simulink model "Subsystem"  (R2020b)
settings: Solver=FixedStepAuto  StartTime=0.0  StopTime=10.0  FixedStep=0.001  RelTol=1e-3
values from neighbouring files (symbols this model uses):
  a0 = 1    [Initializing_prob7.m]
  a1 = 1    [Initializing_prob7.m]
  a2 = -1    [Initializing_prob7.m]
  b0 = 1    [Initializing_prob7.m]
  b1 = 2    [Initializing_prob7.m]
  b2 = -1    [Initializing_prob7.m]
settings Model: Creator=Lakshmi  LastModifiedBy=Lakshmi
settings DataIOCC: SaveOutput=off  SaveTime=off

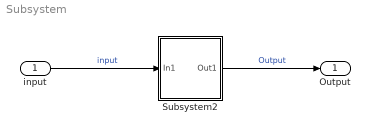
== system Subsystem ==
  input : Inport  OutDataTypeStr=double  PortDimensions=1  SampleTime=[0.001,0]
  Subsystem2 : Subsystem
  Output : Outport  OutDataTypeStr=double  PortDimensions=1  SampleTime=[0.001,0]
  wires:
  input/1 -> Subsystem2/1(In1)  "input"
  Subsystem2/1(Out1) -> Output/1  "Output"

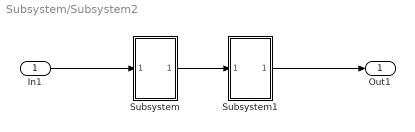
== system Subsystem/Subsystem2 ==
  In1 : Inport
  Subsystem : Subsystem
  Subsystem1 : Subsystem
  Out1 : Outport
  wires:
  In1/1 -> Subsystem/1(In1)
  Subsystem1/1(Out1) -> Out1/1
  Subsystem/1(Out1) -> Subsystem1/1(In1)

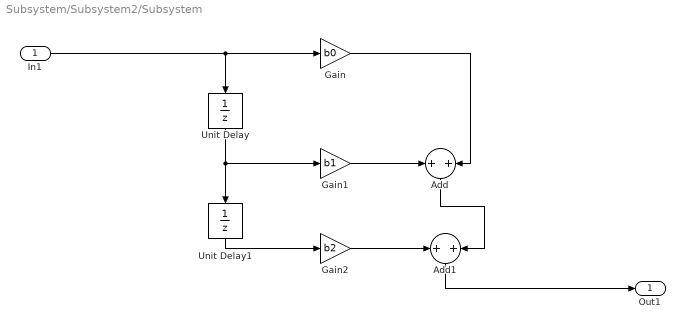
== system Subsystem/Subsystem2/Subsystem ==
  In1 : Inport
  Add : Sum
  Add1 : Sum
  Gain : Gain  Gain=b0
  Gain1 : Gain  Gain=b1
  Gain2 : Gain  Gain=b2
  Unit Delay : UnitDelay  SampleTime=-1  HasFrameUpgradeWarning=on
  Unit Delay1 : UnitDelay  SampleTime=-1  HasFrameUpgradeWarning=on
  Out1 : Outport
  wires:
  Add1/1 -> Out1/1
  Gain/1 -> Add/2
  In1/1 -> Gain/1, Unit Delay/1
  Gain2/1 -> Add1/1
  Gain1/1 -> Add/1
  Add/1 -> Add1/2
  Unit Delay/1 -> Gain1/1, Unit Delay1/1
  Unit Delay1/1 -> Gain2/1

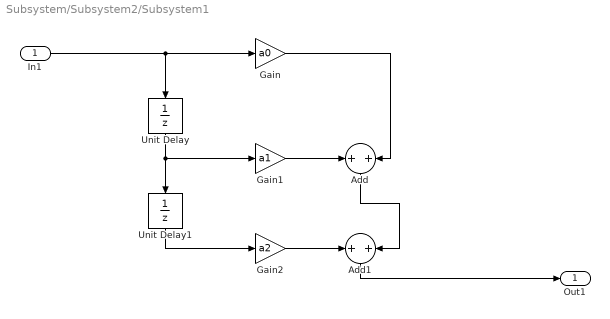
== system Subsystem/Subsystem2/Subsystem1 ==
  In1 : Inport
  Add : Sum
  Add1 : Sum
  Gain : Gain  Gain=a0
  Gain1 : Gain  Gain=a1
  Gain2 : Gain  Gain=a2
  Unit Delay : UnitDelay  SampleTime=-1  HasFrameUpgradeWarning=on
  Unit Delay1 : UnitDelay  SampleTime=-1  HasFrameUpgradeWarning=on
  Out1 : Outport
  wires:
  In1/1 -> Gain/1, Unit Delay/1
  Add1/1 -> Out1/1
  Unit Delay/1 -> Unit Delay1/1, Gain1/1
  Gain2/1 -> Add1/1
  Gain/1 -> Add/2
  Add/1 -> Add1/2
  Gain1/1 -> Add/1
  Unit Delay1/1 -> Gain2/1
